simulink model "mg374610"  (Simulink 7.3)
settings: Solver=FixedStepDiscrete  StartTime=0.0  StopTime=10.0  RelTol=1e-3
libraries: vxlib1 x1, simulink x1
settings Model: Creator=y_amano  LastModifiedBy=dpaul
settings DataIOCC: LimitDataPoints=off  SaveOutput=off  SignalLogging=off  SaveTime=off
settings OptimizationCC: InlineParams=on  InlineInvariantSignals=on  StateBitsets=on  DataBitsets=on  UseTempVars=on  ZeroExternalMemoryAtStartup=off  ZeroInternalMemoryAtStartup=off  NoFixptDivByZeroProtection=on  EfficientFloat2IntCast=on  OptimizeModelRefInitCode=on  LifeSpan=1
settings DebuggingCC: SignalInfNanChecking=warning  SaveWithParameterizedLinksMsg=none  StrictBusMsg=ErrorLevel1
settings HardwareCC: ProdHWDeviceType=32-bit Embedded Processor
settings RTWCC: SystemTargetFile=ert.tlc  GenCodeOnly=on  TemplateMakefile=ert_default_tmf  Description=Real-Time Workshop Embedded Coder (no auto configuration)  ProcessScript=ert_make_rtw_hook
settings CodeAppCC: GenerateComments=off  IgnoreCustomStorageClasses=off  SimulinkBlockComments=off
settings ERTTargetCC: TargetFcnLib=ansi_tfl_tmw.mat  MultiwordLength=2048  IncludeMdlTerminateFcn=off  SuppressErrorStatus=on  SupportAbsoluteTime=off  SupportNonFinite=off  SupportComplex=off  InlinedParameterPlacement=NonHierarchical  ERTCustomFileTemplate=example_file_process.tlc

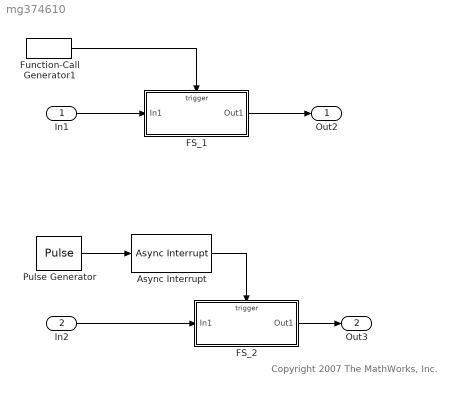
== system mg374610 ==
  note: Copyright 2007 The MathWorks, Inc.
  In1 : Inport  DataType=int32  OutDataType=sfix(16)  OutScaling=2^0  OutDataTypeStr=int32
  In2 : Inport  Port=2  DataType=int32  OutDataType=sfix(16)  OutScaling=2^0  OutDataTypeStr=int32
  Async Interrupt : vxlib1/Async Interrupt  irqnumbers=[1 ]  irqoffsets=[192 ]  irqpriorities=[10 ]  irqpreempts=[0 ]  manageowntimer=on  tickres=1/60  ticklen=32bits  showinput=on
  FS_1 : Subsystem  TreatAsAtomicUnit=on
  FS_2 : Subsystem  TreatAsAtomicUnit=on
  Function-Call Generator1 : simulink/Ports & Subsystems/Function-Call Generator  sample_time=1  numberOfIterations=1
  Pulse Generator : DiscretePulseGenerator  Amplitude=1  Period=2  PulseWidth=1  PhaseDelay=0  SampleTime=1
  Out2 : Outport  OutDataType=sfix(16)  OutScaling=2^0
  Out3 : Outport  Port=2  OutDataType=sfix(16)  OutScaling=2^0
  wires:
  Function-Call Generator1/1 -> FS_1/Trigger
  FS_1/1(Out1) -> Out2/1
  In1/1 -> FS_1/1(In1)
  Async Interrupt/1 -> FS_2/Trigger
  FS_2/1(Out1) -> Out3/1
  Pulse Generator/1 -> Async Interrupt/1
  In2/1 -> FS_2/1(In1)

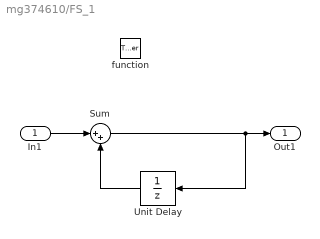
== system mg374610/FS_1 ==
  In1 : Inport  DataType=int32  OutDataType=sfix(16)  OutScaling=2^0  OutDataTypeStr=int32
  function : TriggerPort  TriggerType=function-call
  Sum : Sum  Inputs=|++  OutDataType=sfix(16)  OutScaling=2^0
  Unit Delay : UnitDelay  SampleTime=-1
  Out1 : Outport  OutDataType=sfix(16)  OutScaling=2^0
  wires:
  Unit Delay/1 -> Sum/2
  Sum/1 -> Unit Delay/1, Out1/1
  In1/1 -> Sum/1

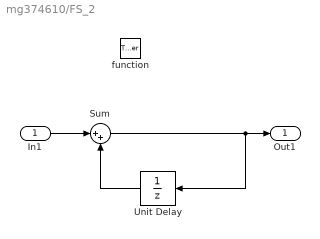
== system mg374610/FS_2 ==
  In1 : Inport  DataType=int32  OutDataType=sfix(16)  OutScaling=2^0  OutDataTypeStr=int32
  function : TriggerPort  TriggerType=function-call
  Sum : Sum  Inputs=|++  OutDataType=sfix(16)  OutScaling=2^0
  Unit Delay : UnitDelay  SampleTime=-1
  Out1 : Outport  OutDataType=sfix(16)  OutScaling=2^0
  wires:
  In1/1 -> Sum/1
  Sum/1 -> Out1/1, Unit Delay/1
  Unit Delay/1 -> Sum/2
